simulink model "b28"  (R2017b)
settings: Solver=VariableStepAuto  StartTime=0.0  StopTime=100  RelTol=1e-3
settings Model: Creator=messi  LastModifiedBy=messi

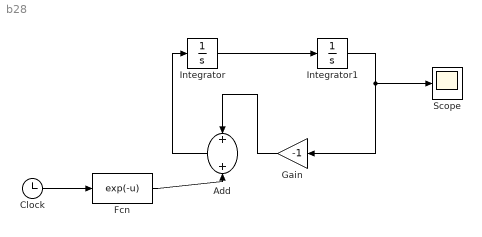
== system b28 ==
  Add : Sum
  Clock : Clock
  Fcn : Fcn  Expr=exp(-u)
  Gain : Gain  Gain=-1
  Integrator : Integrator
  Integrator1 : Integrator  InitialCondition=1
  Scope : Scope
  wires:
  Integrator/1 -> Integrator1/1
  Integrator1/1 -> Scope/1, Gain/1
  Clock/1 -> Fcn/1
  Fcn/1 -> Add/2
  Gain/1 -> Add/1
  Add/1 -> Integrator/1
